simulink model "Thumb_IndexFinger_Control"  (Simulink 6.6)
settings: Solver=ode3  StartTime=0.0  StopTime=10.0  FixedStep=0.01  RelTol=1e-3
libraries: dspmtrx3 x2, dspinverses x1
settings Model: Creator=Jadav Das  LastModifiedBy=Jadav Das

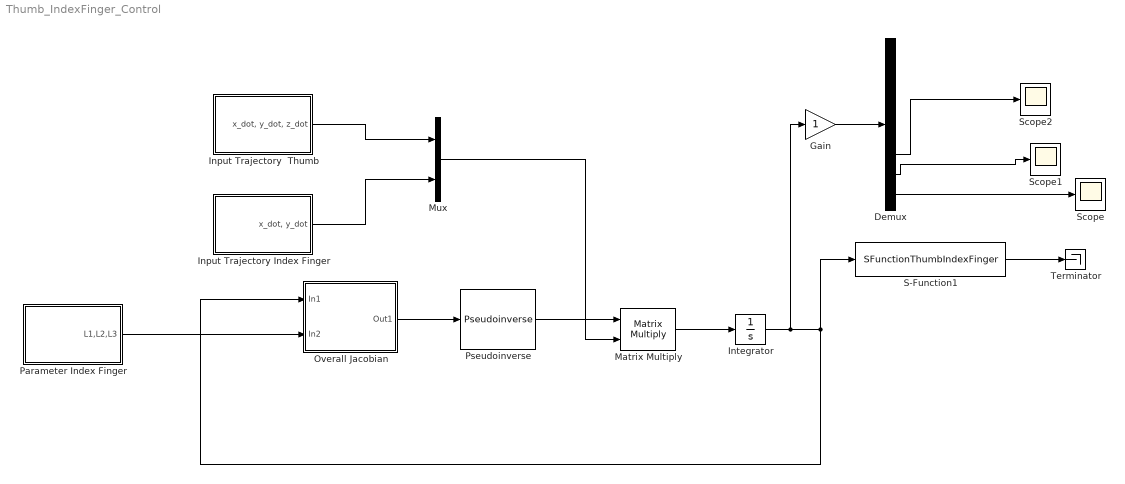
== system Thumb_IndexFinger_Control ==
  Demux : Demux  Outputs=8
  Gain : Gain
  "Input Trajectory Index Finger " : Subsystem
  Input Trajectory  Thumb : Subsystem
  Integrator : Integrator
  Matrix Multiply : Product  Multiplication=Matrix(*)
  Mux : Mux  Inputs=2
  Overall Jacobian : Subsystem
  Parameter Index Finger : Subsystem
  Pseudoinverse : dspinverses/Pseudoinverse  wanterr=off
  S-Function1 : S-Function  FunctionName=SFunctionThumbIndexFinger
  Scope : Scope
  Scope1 : Scope
  Scope2 : Scope
      settings: SaveName=ScopeData2
  Terminator : Terminator
  wires:
  Overall Jacobian/1(Out1) -> Pseudoinverse/1
  Pseudoinverse/1 -> Matrix Multiply/1
  Matrix Multiply/1 -> Integrator/1
  Integrator/1 -> S-Function1/1, Overall Jacobian/1(In1), Gain/1
  Input Trajectory  Thumb/1("x_dot, y_dot, z_dot") -> Mux/1
  "Input Trajectory Index Finger "/1("x_dot, y_dot") -> Mux/2
  Mux/1 -> Matrix Multiply/2
  Parameter Index Finger/1(L1,L2,L3) -> Overall Jacobian/2(In2)
  S-Function1/1 -> Terminator/1
  Demux/8 -> Scope/1
  Demux/7 -> Scope1/1
  Demux/6 -> Scope2/1
  Gain/1 -> Demux/1

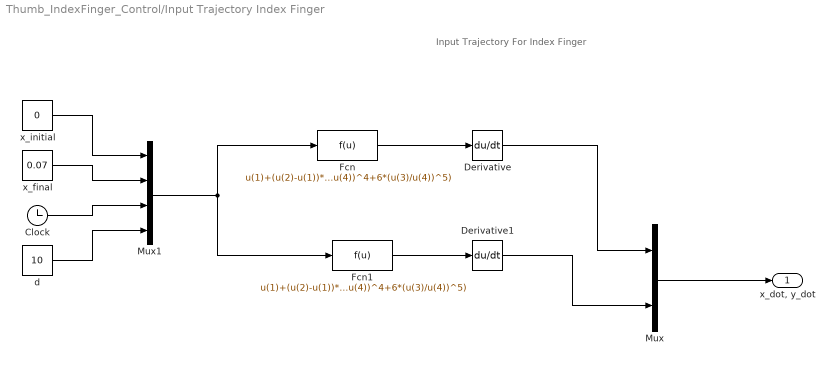
== system Thumb_IndexFinger_Control/Input Trajectory Index Finger  ==
  note: Input Trajectory For Index Finger
  Clock : Clock
      settings: Decimation=10
  Derivative : Derivative
  Derivative1 : Derivative
  Fcn : Fcn  Expr=u(1)+(u(2)-u(1))*(10*(u(3)/u(4))^3-15*(u(3)/u(4))^4+6*(u(3)/u(4))^5)
  Fcn1 : Fcn  Expr=u(1)+(u(2)-u(1))*(10*(u(3)/u(4))^3-15*(u(3)/u(4))^4+6*(u(3)/u(4))^5)
  Mux : Mux  Inputs=2
  Mux1 : Mux
  d : Constant  Value=10
  x_final : Constant  Value=0.07
  x_initial : Constant  Value=0
  "x_dot, y_dot" : Outport
  wires:
  Derivative1/1 -> Mux/2
  Derivative/1 -> Mux/1
  Fcn/1 -> Derivative/1
  Mux/1 -> "x_dot, y_dot"/1
  x_initial/1 -> Mux1/1
  x_final/1 -> Mux1/2
  Clock/1 -> Mux1/3
  d/1 -> Mux1/4
  Mux1/1 -> Fcn/1, Fcn1/1
  Fcn1/1 -> Derivative1/1

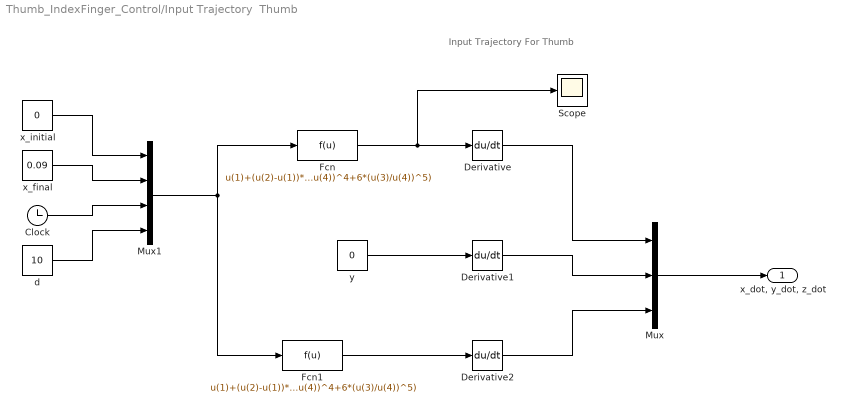
== system Thumb_IndexFinger_Control/Input Trajectory  Thumb ==
  note: Input Trajectory For Thumb
  Clock : Clock
      settings: Decimation=10
  Derivative : Derivative
  Derivative1 : Derivative
  Derivative2 : Derivative
  Fcn : Fcn  Expr=u(1)+(u(2)-u(1))*(10*(u(3)/u(4))^3-15*(u(3)/u(4))^4+6*(u(3)/u(4))^5)
  Fcn1 : Fcn  Expr=u(1)+(u(2)-u(1))*(10*(u(3)/u(4))^3-15*(u(3)/u(4))^4+6*(u(3)/u(4))^5)
  Mux : Mux  Inputs=3
  Mux1 : Mux
  Scope : Scope
      settings: SaveName=ScopeData3
  d : Constant  Value=10
  x_final : Constant  Value=0.09
  x_initial : Constant  Value=0
  y : Constant  Value=0
  "x_dot, y_dot, z_dot" : Outport
  wires:
  Mux/1 -> "x_dot, y_dot, z_dot"/1
  Derivative/1 -> Mux/1
  Derivative1/1 -> Mux/2
  Derivative2/1 -> Mux/3
  x_initial/1 -> Mux1/1
  x_final/1 -> Mux1/2
  Clock/1 -> Mux1/3
  d/1 -> Mux1/4
  Mux1/1 -> Fcn/1, Fcn1/1
  Fcn/1 -> Derivative/1, Scope/1
  y/1 -> Derivative1/1
  Fcn1/1 -> Derivative2/1

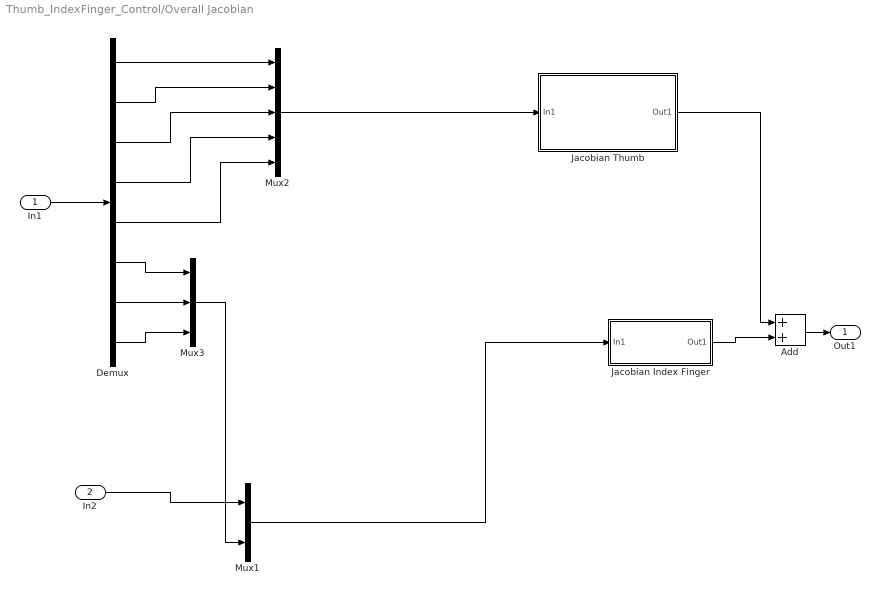
== system Thumb_IndexFinger_Control/Overall Jacobian ==
  In1 : Inport
  In2 : Inport  Port=2
  Add : Sum  OutScaling=2^-10
  Demux : Demux  Outputs=8
  Jacobian Index Finger : Subsystem
  Jacobian Thumb : Subsystem
  Mux1 : Mux  Inputs=2
  Mux2 : Mux  Inputs=5
  Mux3 : Mux  Inputs=3
  Out1 : Outport
  wires:
  Jacobian Index Finger/1(Out1) -> Add/2
  Mux1/1 -> Jacobian Index Finger/1(In1)
  Jacobian Thumb/1(Out1) -> Add/1
  Add/1 -> Out1/1
  In1/1 -> Demux/1
  Demux/1 -> Mux2/1
  Demux/2 -> Mux2/2
  Demux/3 -> Mux2/3
  Demux/4 -> Mux2/4
  Demux/5 -> Mux2/5
  Mux2/1 -> Jacobian Thumb/1(In1)
  In2/1 -> Mux1/1
  Demux/6 -> Mux3/1
  Demux/7 -> Mux3/2
  Demux/8 -> Mux3/3
  Mux3/1 -> Mux1/2

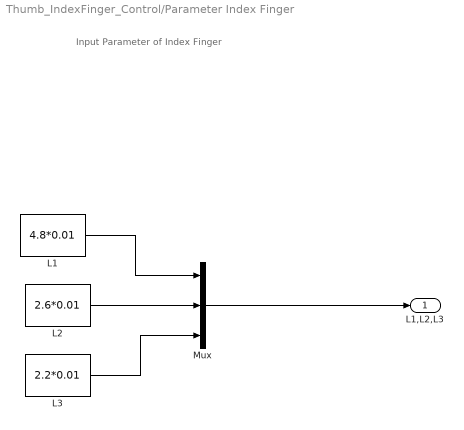
== system Thumb_IndexFinger_Control/Parameter Index Finger ==
  note: Input Parameter of Index Finger
  L1 : Constant  Value=4.8*0.01
  L2 : Constant  Value=2.6*0.01
  L3 : Constant  Value=2.2*0.01
  Mux : Mux  Inputs=3
  L1,L2,L3 : Outport
  wires:
  L1/1 -> Mux/1
  L2/1 -> Mux/2
  L3/1 -> Mux/3
  Mux/1 -> L1,L2,L3/1

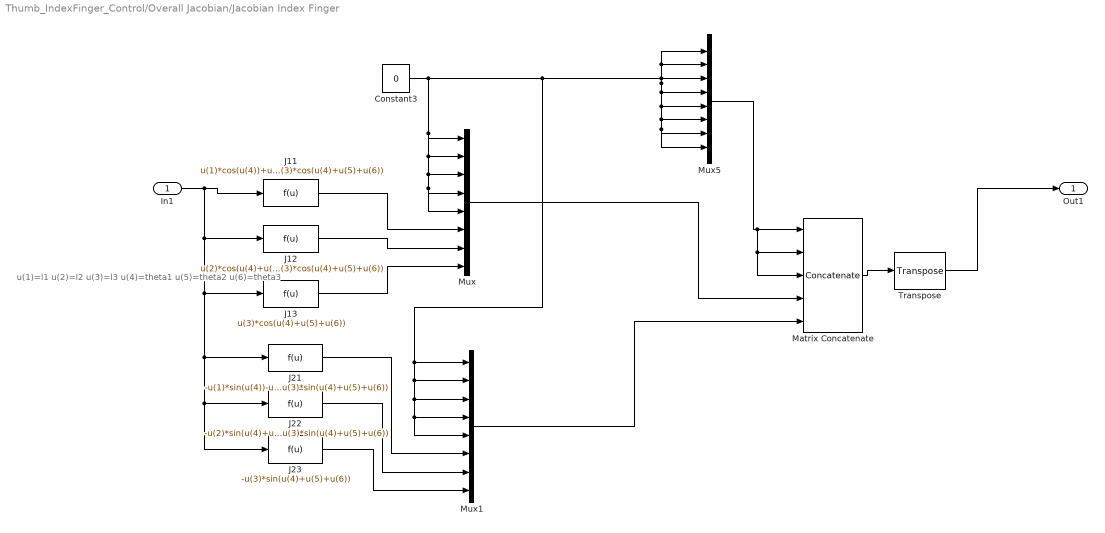
== system Thumb_IndexFinger_Control/Overall Jacobian/Jacobian Index Finger ==
  note: u(1)=l1
      | u(2)=l2
      | u(3)=l3
      | u(4)=theta1
      | u(5)=theta2
      | u(6)=theta3
  In1 : Inport
  Constant3 : Constant  Value=0
  J11 : Fcn  Expr=u(1)*cos(u(4))+u(2)*cos(u(4)+u(5))+u(3)*cos(u(4)+u(5)+u(6))
  J12 : Fcn  Expr=u(2)*cos(u(4)+u(5))+u(3)*cos(u(4)+u(5)+u(6))
  J13 : Fcn  Expr=u(3)*cos(u(4)+u(5)+u(6))
  J21 : Fcn  Expr=-u(1)*sin(u(4))-u(2)*sin(u(4)+u(5))-u(3)*sin(u(4)+u(5)+u(6))
  J22 : Fcn  Expr=-u(2)*sin(u(4)+u(5))-u(3)*sin(u(4)+u(5)+u(6))
  J23 : Fcn  Expr=-u(3)*sin(u(4)+u(5)+u(6))
  Matrix Concatenate : Concatenate  NumInputs=5  Mode=Multidimensional array  ConcatenateDimension=2
  Mux : Mux  Inputs=8
  Mux1 : Mux  Inputs=8
  Mux5 : Mux  Inputs=8
  Transpose : dspmtrx3/Transpose  SystemSampleTime=-1  Hermitian=off  overflowFlag=off
  Out1 : Outport
  wires:
  In1/1 -> J11/1, J12/1, J13/1, J21/1, J22/1, J23/1
  Matrix Concatenate/1 -> Transpose/1
  Transpose/1 -> Out1/1
  J13/1 -> Mux/8
  Constant3/1 -> Mux/1, Mux/2, Mux/3, Mux/4, Mux/5, Mux5/1, Mux5/2, Mux5/3, Mux5/4, Mux5/5, Mux5/6, Mux5/7, Mux5/8, Mux1/1, Mux1/2, Mux1/3, Mux1/4, Mux1/5
  Mux5/1 -> Matrix Concatenate/1, Matrix Concatenate/2, Matrix Concatenate/3
  J11/1 -> Mux/6
  J12/1 -> Mux/7
  J21/1 -> Mux1/6
  J22/1 -> Mux1/7
  J23/1 -> Mux1/8
  Mux/1 -> Matrix Concatenate/4
  Mux1/1 -> Matrix Concatenate/5

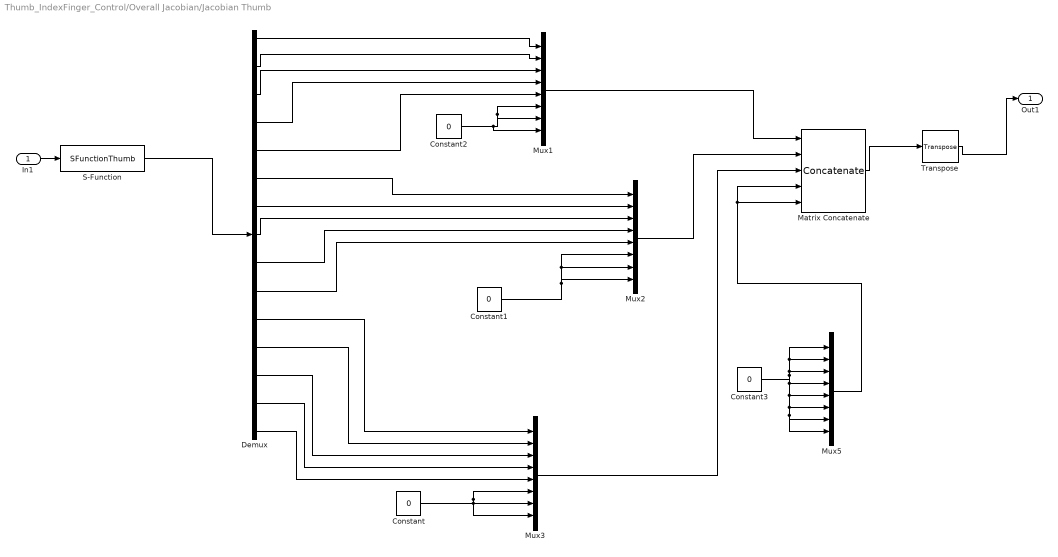
== system Thumb_IndexFinger_Control/Overall Jacobian/Jacobian Thumb ==
  In1 : Inport
  Constant{,1..3} (4 alike) : Constant  Value=0
  Demux : Demux  Outputs=15
  Matrix Concatenate : Concatenate  NumInputs=5  Mode=Multidimensional array  ConcatenateDimension=2
  Mux{1..3,5} (4 alike) : Mux  Inputs=8
  S-Function : S-Function  FunctionName=SFunctionThumb
  Transpose : dspmtrx3/Transpose  SystemSampleTime=-1  Hermitian=off  overflowFlag=off
  Out1 : Outport
  wires:
  S-Function/1 -> Demux/1
  Demux/1 -> Mux1/1
  Demux/2 -> Mux1/2
  Demux/3 -> Mux1/3
  Demux/4 -> Mux1/4
  Demux/5 -> Mux1/5
  Mux1/1 -> Matrix Concatenate/1
  Mux2/1 -> Matrix Concatenate/2
  Mux3/1 -> Matrix Concatenate/3
  Matrix Concatenate/1 -> Transpose/1
  Demux/6 -> Mux2/1
  Demux/7 -> Mux2/2
  Demux/8 -> Mux2/3
  Demux/9 -> Mux2/4
  Demux/10 -> Mux2/5
  Demux/11 -> Mux3/1
  Demux/12 -> Mux3/2
  Demux/13 -> Mux3/3
  Demux/14 -> Mux3/4
  Demux/15 -> Mux3/5
  Transpose/1 -> Out1/1
  In1/1 -> S-Function/1
  Constant/1 -> Mux3/6, Mux3/7, Mux3/8
  Constant1/1 -> Mux2/6, Mux2/7, Mux2/8
  Constant2/1 -> Mux1/6, Mux1/7, Mux1/8
  Constant3/1 -> Mux5/1, Mux5/2, Mux5/3, Mux5/4, Mux5/5, Mux5/6, Mux5/7, Mux5/8
  Mux5/1 -> Matrix Concatenate/4, Matrix Concatenate/5
